simulink model "fuzzyneuro"  (R2021b)
settings: Solver=ode45  StartTime=0.0  StopTime=1  RelTol=1e-3  EnableMultiTasking=on
libraries: spsDistributedParametersLineLib x2, fuzblock x1, spsGroundLib x1, spsSequenceAnalyzerLib x1, spsThreePhaseSeriesRLCBranchLib x1, spsThreePhaseVIMeasurementLib x1, spsThreePhaseFaultLib x1, spsThreePhaseSourceLib x1, spspowerguiLib x1
settings Model: Creator=SAI KUMAR  LastModifiedBy=SAI KUMAR
settings SolverCC: AlgebraicLoopSolver=TrustRegion
settings DataIOCC: LimitDataPoints=on  SaveFormat=Array  ReturnWorkspaceOutputs=off
settings OptimizationCC: LifeSpan=inf
settings DebuggingCC: UnderspecifiedInitializationDetection=Classic  MergeDetectMultiDrivingBlocksExec=none  SolverPrmCheckMsg=warning  SFUnexpectedBacktrackingDiag=warning  SFNoUnconditionalDefaultTransitionDiag=warning  SFExecutionAtInitializationDiag=none  SFMachineParentedDataDiag=warning  ArithmeticOperatorsInVariantConditions=warning
settings HardwareCC: ProdBitPerPointer=32  ProdBitPerSizeT=32  ProdBitPerPtrDiffT=32  ProdLargestAtomicFloat=None  ProdIntDivRoundTo=Undefined  ProdEndianess=Unspecified  ProdWordSize=32  ProdHWDeviceType=32-bit Generic
settings ModelReferenceCC: PropagateSignalLabelsOutOfModel=off
settings SFSimCC: SimUseLocalCustomCode=off  CustomCodeUndefinedFunction=UseInterfaceOnly
settings RTWCC: RTWUseLocalCustomCode=off
settings CodeAppCC: StateflowObjectComments=on
settings GRTTargetCC: TargetLangStandard=C89/C90 (ANSI)
settings ConfigComp: CovMetricSettings=dw  CovSaveCumulativeToWorkspaceVar=on  CovSaveSingleToWorkspaceVar=on  CovExternalEMLEnable=off
settings SimscapeCC: SimscapeNormalizeSystem=off

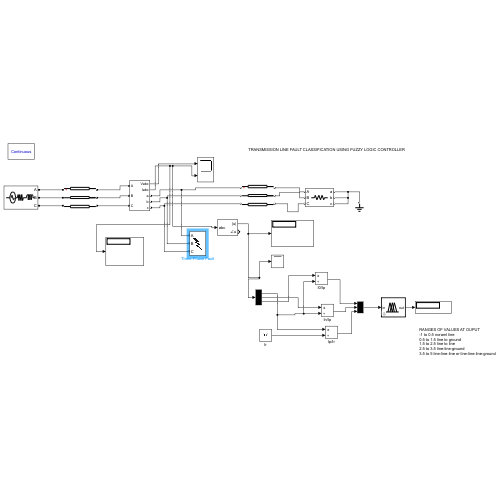
[thumbnail: Simulink's stored preview of the top-level diagram]
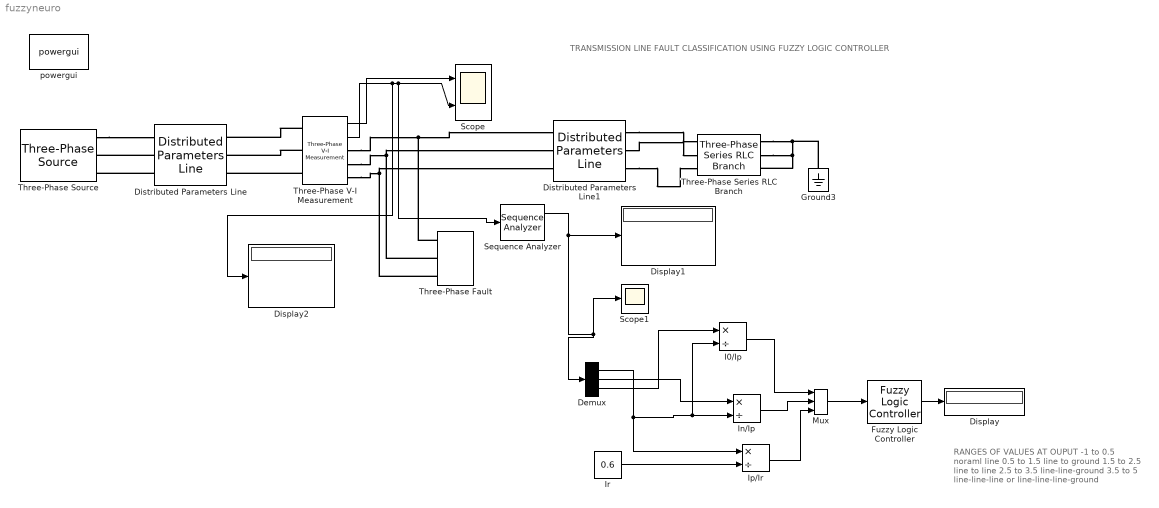
== system fuzzyneuro ==
  note: TRANSMISSION LINE FAULT CLASSIFICATION USING FUZZY LOGIC CONTROLLER
  note: RANGES OF VALUES AT OUPUT
      | -1 to 0.5 noraml line
      | 0.5 to 1.5 line to ground
      | 1.5 to 2.5 line to line
      | 2.5 to 3.5 line-line-ground
      | 3.5 to 5 line-line-line or line-line-line-ground
  Demux : Demux  Outputs=3
  Display : Display
  Display1 : Display
  Display2 : Display
  Distributed Parameters Line : spsDistributedParametersLineLib/Distributed Parameters Line  Phases=3  Length=100  Frequency=50  Resistance=[0.01273 0.3864]  Inductance="[0.9337e-3  4.1264e-3]"  Capacitance=[12.74e-9 7.751e-9]  x1=[0 2.12180139124018e-13 162.503163352374 -377.954852839248;0.000113108313399149 1.07221754004189e-13 175.828011373519 -371.943086104177;0.000226216626798297 2.12799776878164e-15 188.930870542955 -365.461728557379;0.000339324940197446 -1.02968445136273e-13 201.795198054797 -358.51896313346;0.000452433253596594 -2.07934886873029e-13 214.404752257502 -351.123555310186;0.000565541566995743 -3.12638803734444e-13 226.743613159505 -343.284842041763]  x2=[0 -2.48659590939249e-14 138.135927551968 -369.734647040903;0.000113108313399149 -1.39906818492812e-13 151.1841222765 -364.593753202915;0.000226216626798297 -2.54771040769202e-13 164.04144189849 -358.992547336248;0.000339324940197446 -3.69313605931078e-13 176.691653614092 -352.938101154043;0.000452433253596594 -4.83389900089484e-13 189.118786100248 -346.438058600772;0.000565541566995743 -5.96855898038484e-13 201.30714967902 -339.500626201502]  x3=[0 2.1451652340325e-15 0.766337670225195 -0.582740927008281;0.000113108313399149 1.95846312149355e-15 0.786556679557863 -0.55514773048222;0.000226216626798297 1.76928838257352e-15 0.805782634298516 -0.526853641042362;0.000339324940197446 1.57787985682213e-15 0.823991261024606 -0.497894380940103;0.000452433253596594 1.38447920402105e-15 0.841159570724846 -0.468306512227454;0.000565541566995743 1.18933059908018e-15 0.857265887823618 -0.438127390596197]  x4=[0 -7.63223278501858e-16 0.190847877720396 -2.22947369148662;0.000113108313399149 -8.29076218758218e-16 0.269932904026569 -2.22128613212822;0.000226216626798297 -8.93882422056434e-16 0.34867713084957 -2.21029412338808;0.000339324940197446 -9.57560068358042e-16 0.42698114092161 -2.19651154305154;0.000452433253596594 -1.02002876246621e-15 0.504746072763542 -2.1799557920956;0.000565541566995743 -1.08120963552744e-15 0.58187374550084 -2.16064777271961]  x5=0.000565541566995743  V1=ones(3,3)  V2=ones(3,3)  I1=ones(3,3)  I2=ones(3,3)  nHarmo=1  Measurements=None  Decoupling=off  VsMag0=0  VrMag0=0  VsAngle0=0  VrAngle0=0  IsMag0=0  IrMag0=0  IsAngle0=0  IrAngle0=0
      settings: SourceProductBaseCode=PS
  Distributed Parameters Line1 : spsDistributedParametersLineLib/Distributed Parameters Line  Phases=3  Length=1000  Frequency=50  Resistance=[0.01273 0.3864]  Inductance="[0.9337e-3  4.1264e-3]"  Capacitance=[12.74e-9 7.751e-9]  x1=[0 3.23801906680303e-12 -228.567622049186 -321.779560963533;0.00113108313399149 3.05889552167155e-12 -102.338457742084 -381.198221100355;0.00226216626798297 2.49758236327602e-12 36.677248409741 -392.988578908082;0.00339324940197446 1.62421211409304e-12 171.110364771886 -355.677503886225;0.00452433253596594 5.47906852796675e-13 284.164325267373 -273.926778443514;0.00565541566995743 -5.96855898038484e-13 361.713753879395 -157.950637724513]  x2=[0 4.67488157249352e-14 -147.176499973282 61.4799346018603;0.00113108313399149 1.83596456133649e-13 -159.37156009973 6.43508620085768;0.00226216626798297 2.97504882676038e-13 -151.654153622377 -49.413785446118;0.00339324940197446 3.7424195921691e-13 -124.988521580539 -99.0887177036094;0.00452433253596594 4.04219874273859e-13 -82.7063657356233 -136.383142542764;0.00565541566995743 3.83693077310454e-13 -30.0905735467962 -156.637357889679]  x3=[0 1.91140440533446e-15 0.0630518076941966 -0.928160658705875;0.00113108313399149 2.08205188763171e-15 0.382028641350819 -0.848240447049347;0.00226216626798297 1.9925601791354e-15 0.653273416929867 -0.662337966264659;0.00339324940197446 1.65411070177323e-15 0.842895818418911 -0.393680553386554;0.00452433253596594 1.10899057321433e-15 0.927203728261842 -0.0758352498523585;0.00565541566995743 4.2530909946158e-16 0.895663407326451 0.251485187633787]  x4=[0 8.48307311879621e-17 -1.96241042833227 0.819756311760227;0.00113108313399149 1.3856897097362e-15 -2.12501596094533 0.0858036457591576;0.00226216626798297 2.51341553923898e-15 -2.02211421403882 -0.658869642099378;0.00339324940197446 3.32710602294195e-15 -1.66656210886935 -1.3212213429925;0.00452433253596594 3.72509569071715e-15 -1.10278362808271 -1.818494808772;0.00565541566995743 3.65765825536959e-15 -0.401219320567155 -2.08855887077708]  x5=0.00565541566995743  V1=ones(3,3)  V2=ones(3,3)  I1=ones(3,3)  I2=ones(3,3)  nHarmo=1  Measurements=Phase-to-ground voltages  Decoupling=off  VsMag0=0  VrMag0=0  VsAngle0=0  VrAngle0=0  IsMag0=0  IrMag0=0  IsAngle0=0  IrAngle0=0
      settings: SourceProductBaseCode=PS
  Fuzzy Logic Controller : fuzblock/Fuzzy Logic  Controller  FIS='member.fis'  OutputSampleNumber=101  DataType=double  FuzzifiedInputs=off  RuleFiringStrengths=off  RuleOutputs=off  AggregatedOutputs=off  SimulateUsing=Interpreted execution  OutOfRangeInputValueMessage=warning  NoRuleFiredMessage=warning  EmptyOutputFuzzySetMessage=warning
  Ground3 : spsGroundLib/Ground  LConnTagsString=a
  I0/Ip : Product  Inputs=*/
  In/Ip : Product  Inputs=*/
  Ip/Ir : Product  Inputs=*/
  Ir : Constant  Value=0.6
  Mux : Mux  Inputs=3
  Scope : Scope  NumInputPorts=2
  Scope1 : Scope
  Sequence Analyzer : spsSequenceAnalyzerLib/Sequence Analyzer  Freq=50  n=1  seq=Positive Negative Zero  InInit=[1, 0]  Ts=0
      settings: SourceProductBaseCode=PS
  Three-Phase Series RLC Branch : spsThreePhaseSeriesRLCBranchLib/Three-Phase Series RLC Branch  LConnTagsString=A|B|C  RConnTagsString=A|B|C  BranchType=R  Resistance=100  Inductance=1e-3  Capacitance=1e-6  Measurements=None
  Three-Phase V-I Measurement : spsThreePhaseVIMeasurementLib/Three-Phase V-I Measurement  VoltageMeasurement=phase-to-phase  SetLabelV=off  LabelV=Vabc  Vpu=off  VpuLL=off  CurrentMeasurement=yes  SetLabelI=off  LabelI=Iabc  Ipu=off  Pbase=100e6  Vbase=500e3  OutputType=Complex  PhasorSimulation=off  PSBequivalent=0
  Three-Phase Fault : spsThreePhaseFaultLib/Three-Phase Fault  InitialStates=0  FaultA=on  FaultB=on  FaultC=off  GroundFault=off  SwitchTimes=[ 25/50 100/50]  External=off  SwitchStatus=NaN  FaultResistance=0.001  GroundResistance=0.001  SnubberResistance=1e6  SnubberCapacitance=inf  Measurements=None
  Three-Phase Source : spsThreePhaseSourceLib/Three-Phase Source  InternalConnection=Y  VoltagePhases=off  Voltage=415  PhaseAngle=0  Voltage_phases=[25e3 25e3 25e3]/sqrt(3)  PhaseAngles_phases=[0 -120 +120]  Frequency=50  NonIdealSource=on  SpecifyImpedance=on  Resistance=0.8929  Inductance=16.58e-3  ShortCircuitLevel=100e6  BaseVoltage=25e3  XRratio=7  BusType=swing  Pref=0  Qref=0  Prefabc=[10e3, 10e3, 10e3]  Qrefabc=[0, 0, 0]  Qmin=-inf  Qmax=inf
  powergui : spspowerguiLib/powergui  Priority=1  SimulationMode=Continuous  SampleTime=50e-6  frequency=60  Iterations=50  frequencyindice=50  Pbase=100e6  ErrMax=1e-4  UnitsV=kV  UnitsW=MW  buscounter=0  FunctionMessages=off  echomessages=off  EnableUseOfTLC=off  CurrentSourceSwitches=on  DisableSnubberDevices=off  DisableRonSwitches=off  DisableVfSwitches=off  DisplayEquations=off  AutomaticDiscreteSolvers=off  SolverType=Tustin  Interpol=off  ExternalGateDelay=off  methode=off  Ts=0  x0status=blocks  SPID=off  SwTol=0  HookPort=off  NonlinearTolerance=1e-4  nMaxIteration=100  ContinueOnMaxIteration=off  RestoreLinks=warning  ResistiveCurrentMeasurement=off  Frange=[0:2:500]  Ylog=off  Xlog=on  ShowGrid=off  save=off  variable=ZData  structure=0  ZoomFFT=off  StartTime=0.0  cycles=1  DisplayStyle=1  fundamental=60  FreqAxis=off  MaxFrequency=1000  frequencyindicesteady=1  RmsSteady=1  display=off
  wires:
  Three-Phase V-I Measurement/1 -> Scope/1
  Sequence Analyzer/1 -> Demux/1, Scope1/1, Display1/1
  I0/Ip/1 -> Mux/1
  In/Ip/1 -> Mux/2
  Ip/Ir/1 -> Mux/3
  Mux/1 -> Fuzzy Logic Controller/1
  Fuzzy Logic Controller/1 -> Display/1
  Demux/3 -> I0/Ip/1
  Demux/1 -> Ip/Ir/1, I0/Ip/2, In/Ip/2
  Demux/2 -> In/Ip/1
  Three-Phase V-I Measurement/2 -> Display2/1, Sequence Analyzer/1, Scope/2
  Ir/1 -> Ip/Ir/2
  connections:
  Three-Phase Source/RConn1 -- Distributed Parameters Line/LConn1
  Distributed Parameters Line/LConn2 -- Three-Phase Source/RConn2
  Distributed Parameters Line/LConn3 -- Three-Phase Source/RConn3
  Three-Phase V-I Measurement/LConn1 -- Distributed Parameters Line/RConn1
  Three-Phase V-I Measurement/LConn2 -- Distributed Parameters Line/RConn2
  Three-Phase V-I Measurement/LConn3 -- Distributed Parameters Line/RConn3
  Three-Phase V-I Measurement/RConn2 -- Distributed Parameters Line1/LConn2 -- Three-Phase Fault/LConn2
  Three-Phase V-I Measurement/RConn1 -- Distributed Parameters Line1/LConn1 -- Three-Phase Fault/LConn1
  Three-Phase V-I Measurement/RConn3 -- Distributed Parameters Line1/LConn3 -- Three-Phase Fault/LConn3
  Distributed Parameters Line1/RConn1 -- Three-Phase Series RLC Branch/LConn1
  Distributed Parameters Line1/RConn2 -- Three-Phase Series RLC Branch/LConn2
  Distributed Parameters Line1/RConn3 -- Three-Phase Series RLC Branch/LConn3
  Three-Phase Series RLC Branch/RConn1 -- Ground3/LConn1 -- Three-Phase Series RLC Branch/RConn2 -- Three-Phase Series RLC Branch/RConn3
